simulink model "small_test"  (R2014b)
settings: Solver=FixedStepDiscrete  SolverMode=SingleTasking  StartTime=0.0  StopTime=20e-6*2  RelTol=1e-3
PreLoadFcn:
  | userName = getenv('UserName');
  | 
  | if strcmp(userName,'Tim')
  | cd C:\MA_1\Sysgen_small_test
  | else
  | cd D:\MA_1\Sysgen_small_test
  | end
InitFcn:
  | userName = getenv('UserName');
  | 
  | if strcmp(userName,'Tim')
  | cd C:\MA_1\Sysgen_small_test
  | else
  | cd D:\MA_1\Sysgen_small_test
  | end
undefined symbols (not defined in the file): bitPerSymb, gcbh, Tb, Ts, usedSubCar, xlBlockLoadCallback
libraries: xbsIndex_r4 x56, commrandsrc2 x1, simulink x1
settings Model: Creator=Tim-UML  LastModifiedBy=Tim-UML
settings DebuggingCC: AssertControl=DisableAll
settings HardwareCC: ProdBitPerLong=64  ProdBitPerPointer=64  ProdWordSize=64  ProdHWDeviceType=Generic->64-bit Embedded Processor (LP64)  TargetHWDeviceType=32-bit Generic

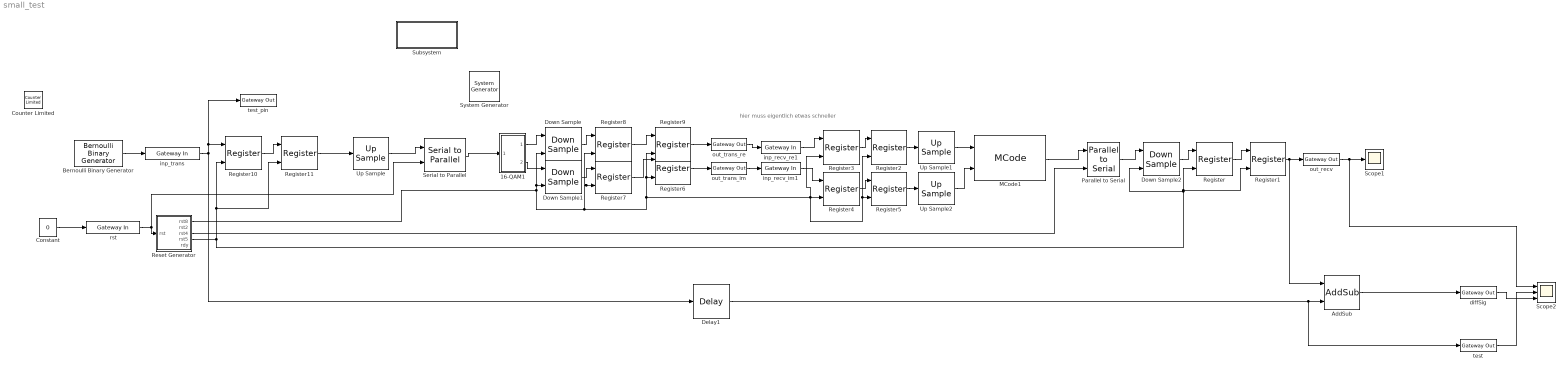
== system small_test ==
  note: hier muss eigentlich etwas schneller
  " System Generator" : xbsIndex_r4/ System Generator  Tag=genX  xilinxfamily=zynq  part=xc7z020  speed=-1  package=clg400  synthesis_tool=Vivado  clock_wrapper=Clock Enables  directory=./netlistFin3  proj_type=Vivado  Synth_file=Vivado Synthesis Defaults  Impl_file=Vivado Implementation Defaults  testbench=on  simulink_period=sysgenSystemPeriod  sysclk_period=1000/250  dcm_input_clock_period=10  incr_netlist=off  trim_vbits=Everywhere in SubSystem  dbl_ovrd=According to Block Masks  core_generation=According to Block Masks  run_coregen=off  deprecated_control=off  eval_field=0  block_type=sysgen
  16-QAM1 : Subsystem
  AddSub : xbsIndex_r4/AddSub  mode=Subtraction  use_carryin=off  use_carryout=off  en=off  latency=1  precision=User Defined  arith_type=Unsigned  n_bits=1  bin_pt=0  quantization=Truncate  overflow=Wrap  use_behavioral_HDL=off  hw_selection=Fabric  pipelined=off  dbl_ovrd=off  block_type=addsub
  Bernoulli Binary Generator : commrandsrc2/Bernoulli Binary Generator  P=0.5  seed=1604198  Ts=Tb  frameBased=off  sampPerFrame=1  orient=off  outDataType=boolean
      settings: AttributesFormatString=|
      | Sample Time= %<Ts>
      | Prob zero=%<P>
  Constant : Constant  Value=0
  Counter Limited : simulink/Sources/Counter Limited  uplimit=1  tsamp=Tb
  Delay1 : xbsIndex_r4/Delay  rst=off  infoeditControl=Selection of Reset will increase slice count due to use of real FFs and instead of SRLs  en=off  latency=14  reg_retiming=off  dbl_ovrd=off  block_type=delay
  Down Sample : xbsIndex_r4/Down Sample  sample_ratio=2  sample_phase="Last Value of Frame  (most efficient)"  en=off  rst=on  latency=1  dbl_ovrd=off  block_type=dsamp
  Down Sample1 : xbsIndex_r4/Down Sample  sample_ratio=2  sample_phase="Last Value of Frame  (most efficient)"  en=off  rst=on  latency=1  dbl_ovrd=off  block_type=dsamp
  Down Sample2 : xbsIndex_r4/Down Sample  sample_ratio=5  sample_phase="Last Value of Frame  (most efficient)"  en=off  rst=on  latency=1  dbl_ovrd=off  block_type=dsamp
  MCode1 : xbsIndex_r4/MCode  mfname=Demod_16QAM  explicit_period=off  period=1  inputsTable={'boundInpExpr'=>['',''],'inputs'=>['I','Q']}  outputsTable={'outputs'=>['y1'],'suppressOut'=>['off']}  enable_stdout=off  enable_debug=off  suppress_output=on  defparams={}  hide_port_list={}  dbl_ovrd=off  block_type=mcode
  Parallel to Serial : xbsIndex_r4/Parallel to Serial  output_order=Most Significant Word First  arith_type=Unsigned  output_bits=1  bin_pt=0  rst=on  en=off  latency=1  dbl_ovrd=off  block_type=p2s
      settings: infoedit=Each sample presented at the input becomes several samples presented serially at the output.
  Register{,1..11} (12 alike) : xbsIndex_r4/Register  init=0  rst=on  en=off  dbl_ovrd=off  block_type=register
  Reset Generator : Subsystem  LoadFcn=xlBlockLoadCallback(gcbh);  mask(Xilinx Reset Generator Block){infoedit=Captures the user's reset signal that is running at the system sample rate, and produces a downsampled reset signal running at the rates specified on the block.  The downsampled reset signals are synchronized in the same way as they are during startup.  The RDY output signal indicates when the downsampled resets are no longer asserted after the input reset is detected., rates=[5 4 2 8], previous_rates=5  4  2  8, has_advanced_control=0, sggui_pos=-1,-1,-1,-1, block_type=resetgenerator, block_version=1.0, sg_icon_stat=55,56,1,5,white,blue,0,4a55d45e49b130f2bb5565f39ca9cc33,right,,[ ],[ ], sg_mask_display=|, sg_list_contents=, sg_blockgui_xml=}
      mask sg_mask_display=|
      | fprintf('','COMMENT: begin icon graphics');
      | patch([0 55 55 0 0 ],[0 0 56 56 0 ],[0.77 0.82 0.91 ]);
      | plot([0 55 55 0 0 ],[0 0 56 56 0 ]);
      | patch([11.425 21.54 28.54 35.54 42.54 28.54 18.425 11.425 ],[35.77 35.77 42.77 35.77 42.77 42.77 42.77 35.77 ],[1 1 1 ]);
      | patch([18.425 28.54 21.54 11.425 18.425 ],[28.77 28.77 35.77 35.77 28.77 ],[0.931 0.946 0.973 ]);
      | patch([11.425 21.54 28.54 18.425 11.425 ],[21.77 21.77 28.77 28.77 21.77 ],[1 1 1 ]);
      | patch([18.425 42.54 35.54 28.54 21.54 11.425 18.425 ],[14.77 14.77 21.77 14.77 21.77 21.77 14.77 ],[0.931 0.946 0.973 ]);
      | fprintf('','COMMENT: end icon graphics');
      | fprintf('','COMMENT: begin icon text');
      | color('black');port_label('input',1,'rst');
      | color('black');port_label('output',1,'rst8');
      | color('black');port_label('output',2,'rst2');
      | color('black');port_label('output',3,'rst4');
      | color('black');port_label('output',4,'rst5');
      | color('black');port_label('output',5,'rdy');
      | fprintf('','COMMENT: end icon text');
      mask prompts: infoedit ""; rates "Specify design sample rates in MATLAB vector format, e.g. [2  4 16]"; previous_rates ""; has_advanced_control ""; sggui_pos ""; block_type ""; block_version ""; sg_icon_stat ""; sg_mask_display ""; sg_list_contents ""; sg_blockgui_xml ""
      mask help: Captures the user's reset signal that is running at the system sample rate, and produces a downsampled reset signal running at the rates specified on the block. The downsampled reset signals are synchronized in the same way as they are during startup. The RDY output signal indicates when the downsampled resets are no longer asserted after the input reset is detected.
      mask init:
      | try
      |   tmp_gcb = gcb;
      |   tmp_gcbh = gcbh;
      |   if (strcmp('SysGenIndex',get_param(bdroot(tmp_gcbh),'tag')) && ~isempty(regexp(bdroot(tmp_gcb), '^xbs', 'once')))
      |     return;
      |   end;
      |   xlMungeMaskParams;
      | 
      |   block_type='resetgenerator';
      | 
      |   serialized_declarations = '{''xinports''=>''DoubleVector'',''xoutports''=>''DoubleVector'',''block_type''=>''String''}';
      |   xlReset_init();
      |   ptable_ = xlblockprep(get_param(tmp_gcb, 'MaskWSVariables'));
      |   try
      |     xlBlockMoveCallback(tmp_gcbh);
      |   catch 
      |      clear global xl_updateicon_recursion_guard;
      |   end;
      | catch
      |   global dbgsysgen;
      |   if(~isempty(dbgsysgen) && dbgsysgen)
      |     e = regexprep(lasterr, '\n', '\nError: ');
      |     disp(['Error: While running MaskInit code on block ' tmp_gcb ': ' e]);
      |     error(e);
      |   end
      | end
      settings: CopyFcn=tmp_gcbh = gcbh;set_param(tmp_gcbh,'linkstatus','none');xlBlockMoveCallback(gcbh);  DeleteFcn=xlDestroyGui(gcbh);  ModelCloseFcn=xlDestroyGui(gcbh);  PreSaveFcn=xlBlockPreSaveCallback(gcbh);  PostSaveFcn=xlBlockPostSaveCallback(gcbh);  DestroyFcn=xlDestroyGui(gcbh);  OpenFcn=xlOpenGui(gcbh, 'xlReset_gui.xml', -1, -1)  CloseFcn=xlDestroyGui(gcbh);  MoveFcn=xlBlockMoveCallback(gcbh);
      mask Help: eval('');xlDoc('-book','sysgen','-topic','Reset_Generator');
      mask Display:
      | fprintf('','COMMENT: begin icon graphics');
      | patch([0 55 55 0 0 ],[0 0 56 56 0 ],[0.77 0.82 0.91 ]);
      | plot([0 55 55 0 0 ],[0 0 56 56 0 ]);
      | patch([11.425 21.54 28.54 35.54 42.54 28.54 18.425 11.425 ],[35.77 35.77 42.77 35.77 42.77 42.77 42.77 35.77 ],[1 1 1 ]);
      | patch([18.425 28.54 21.54 11.425 18.425 ],[28.77 28.77 35.77 35.77 28.77 ],[0.931 0.946 0.973 ]);
      | patch([11.425 21.54 28.54 18.425 11.425 ],[21.77 21.77 28.77 28.77 21.77 ],[1 1 1 ]);
      | patch([18.425 42.54 35.54 28.54 21.54 11.425 18.425 ],[14.77 14.77 21.77 14.77 21.77 21.77 14.77 ],[0.931 0.946 0.973 ]);
      | fprintf('','COMMENT: end icon graphics');
      | fprintf('','COMMENT: begin icon text');
      | color('black');port_label('input',1,'rst');
      | color('black');port_label('output',1,'rst8');
      | color('black');port_label('output',2,'rst2');
      | color('black');port_label('output',3,'rst4');
      | color('black');port_label('output',4,'rst5');
      | color('black');port_label('output',5,'rdy');
      | fprintf('','COMMENT: end icon text');
  Scope1 : Scope
      settings: TimeRange=1.102458307597285e-07  YMin=-0  YMax=2  SaveName=ScopeData92
  Scope2 : Scope  NumInputPorts=3
      settings: TimeRange=1.102458307597285e-07  YMin=-0~-5~-5  YMax=2~5~5
  Serial to Parallel : xbsIndex_r4/Serial to Parallel  input_order=Most Significant Word First  arith_type=Unsigned  output_bits=4  bin_pt=0  rst=on  en=off  latency=1  dbl_ovrd=off  block_type=s2p
      settings: infoedit=Groups of samples presented serially at the input become single samples presented at the output.
  Subsystem : Subsystem  mask(Model Parameters){upsample=No, dmtOfdm=DMT, guardInterval=Yes, AWGN=No, channel=No, equalizer=No, SampleTime=20e-9, BitTime=20e-9, modu_mode=0, radio_precision=fixpoint, bitCount=16, fracLen=13, impulseResponse=No}
      mask prompts: upsample "Enable Upsampling"; dmtOfdm "Select FFT Inputorder"; guardInterval "Guard Interval"; SampleTime "Sample Time [s]"; BitTime "Bit Time"; modu_mode "Modulation Mode"; radio_precision "Select Precision"; bitCount "Bit Count"; fracLen "Fraction Length"; impulseResponse "Measure Impulse Response"
      mask init:
      | initScript
      mask TypeOptions upsample: No | Yes
      mask TypeOptions dmtOfdm: OFDM | DMT
      mask TypeOptions guardInterval: No | Yes
      mask TypeOptions AWGN: No | Yes
      mask TypeOptions channel: No | Yes
      mask TypeOptions equalizer: No | Yes
      mask TypeOptions radio_precision: double | fixpoint
      mask TypeOptions impulseResponse: No | Yes
      mask DialogControl Container3 Prompt: Only for Fixpoint
      mask Display: disp('Edit Model\n Parameters')
  Up Sample : xbsIndex_r4/Up Sample  sample_ratio=5  copy_samples=on  en=off  latency=0  dbl_ovrd=off  block_type=usamp
  Up Sample1 : xbsIndex_r4/Up Sample  sample_ratio=2  copy_samples=on  en=off  latency=0  dbl_ovrd=off  block_type=usamp
  Up Sample2 : xbsIndex_r4/Up Sample  sample_ratio=2  copy_samples=on  en=off  latency=0  dbl_ovrd=off  block_type=usamp
  diffSig : xbsIndex_r4/Gateway Out  inherit_from_input=off  hdl_port=on  rows=1  columns=1  UseAsDAC=off  DACChannel='1'  interface=None  automatic_assignment=on  address_offset=hex2dec('00')  intf_description=''  timing_constraint=Data Rate  locs_specified=off  LOCs={}  io_standard={}  block_type=gatewayout
  inp_recv_im1 : xbsIndex_r4/Gateway In  gui_display_data_type=Fixed-point  arith_type="Signed  (2's comp)"  n_bits=16  bin_pt=fracLen  preci_type=Single  exp_width=8  frac_width=24  rows=1  columns=1  quantization="Round  (unbiased: +/- Inf)"  overflow=Saturate  period=Tb/5*8  UseAsADC=off  ADCChannel='1'  interface=None  automatic_assignment=on  address_offset=hex2dec('00')  intf_description=''  timing_constraint=None  locs_specified=off  LOCs={}  io_standard={}  inherit_from_input=off  hdl_port=on  dbl_ovrd=off  block_type=gatewayin
  inp_recv_re1 : xbsIndex_r4/Gateway In  gui_display_data_type=Fixed-point  arith_type="Signed  (2's comp)"  n_bits=16  bin_pt=fracLen  preci_type=Single  exp_width=8  frac_width=24  rows=1  columns=1  quantization="Round  (unbiased: +/- Inf)"  overflow=Saturate  period=Tb/5*8  UseAsADC=off  ADCChannel='1'  interface=None  automatic_assignment=on  address_offset=hex2dec('00')  intf_description=''  timing_constraint=None  locs_specified=off  LOCs={}  io_standard={}  inherit_from_input=off  hdl_port=on  dbl_ovrd=off  block_type=gatewayin
  inp_trans : xbsIndex_r4/Gateway In  gui_display_data_type=Fixed-point  arith_type=Unsigned  n_bits=1  bin_pt=0  preci_type=Single  exp_width=8  frac_width=24  rows=1  columns=1  quantization=Truncate  overflow=Wrap  period=Tb  UseAsADC=off  ADCChannel='1'  interface=None  automatic_assignment=on  address_offset=hex2dec('00')  intf_description=''  timing_constraint=None  locs_specified=off  LOCs={}  io_standard={}  inherit_from_input=off  hdl_port=on  dbl_ovrd=off  block_type=gatewayin
  out_recv : xbsIndex_r4/Gateway Out  inherit_from_input=off  hdl_port=on  rows=1  columns=1  UseAsDAC=off  DACChannel='1'  interface=None  automatic_assignment=on  address_offset=hex2dec('00')  intf_description=''  timing_constraint=Data Rate  locs_specified=off  LOCs={}  io_standard={}  block_type=gatewayout
  out_trans_im : xbsIndex_r4/Gateway Out  inherit_from_input=on  hdl_port=on  rows=1  columns=1  UseAsDAC=off  DACChannel='1'  interface=None  automatic_assignment=on  address_offset=hex2dec('00')  intf_description=''  timing_constraint=None  locs_specified=off  LOCs={}  io_standard={}  block_type=gatewayout
  out_trans_re : xbsIndex_r4/Gateway Out  inherit_from_input=on  hdl_port=on  rows=1  columns=1  UseAsDAC=off  DACChannel='1'  interface=None  automatic_assignment=on  address_offset=hex2dec('00')  intf_description=''  timing_constraint=None  locs_specified=off  LOCs={}  io_standard={}  block_type=gatewayout
  rst : xbsIndex_r4/Gateway In  gui_display_data_type=Boolean  arith_type=Boolean  n_bits=1  bin_pt=0  preci_type=Single  exp_width=8  frac_width=24  rows=1  columns=1  quantization=Truncate  overflow=Wrap  period=SystemPeriod  UseAsADC=off  ADCChannel='1'  interface=None  automatic_assignment=on  address_offset=hex2dec('00')  intf_description=''  timing_constraint=None  locs_specified=off  LOCs={}  io_standard={}  inherit_from_input=off  hdl_port=on  dbl_ovrd=off  block_type=gatewayin
  test : xbsIndex_r4/Gateway Out  inherit_from_input=off  hdl_port=off  rows=1  columns=1  UseAsDAC=off  DACChannel='1'  interface=None  automatic_assignment=on  address_offset=hex2dec('00')  intf_description=''  timing_constraint=Data Rate  locs_specified=off  LOCs={}  io_standard={}  block_type=gatewayout
  test_pin : xbsIndex_r4/Gateway Out  inherit_from_input=on  hdl_port=on  rows=1  columns=1  UseAsDAC=off  DACChannel='1'  interface=None  automatic_assignment=on  address_offset=hex2dec('00')  intf_description=''  timing_constraint=None  locs_specified=off  LOCs={}  io_standard={}  block_type=gatewayout
  wires:
  out_trans_re/1 -> inp_recv_re1/1
  out_trans_im/1 -> inp_recv_im1/1
  inp_recv_re1/1 -> Register3/1
  inp_recv_im1/1 -> Register4/1
  16-QAM1/1(Out2) -> Down Sample/1
  16-QAM1/2(Out3) -> Down Sample1/1
  MCode1/1 -> Parallel to Serial/1
  Parallel to Serial/1 -> Down Sample2/1
  inp_trans/1 -> test_pin/1, Register10/1, Delay1/1
  Serial to Parallel/1 -> 16-QAM1/1(In1)
  out_recv/1 -> Scope2/1, Scope1/1
  Register/1 -> Register1/1
  Register2/1 -> Up Sample1/1
  Register3/1 -> Register2/1
  Register4/1 -> Register5/1
  Register5/1 -> Up Sample2/1
  Register6/1 -> out_trans_im/1
  Register7/1 -> Register6/1
  Register8/1 -> Register9/1
  Register9/1 -> out_trans_re/1
  Register10/1 -> Register11/1
  Register11/1 -> Up Sample/1
  Up Sample/1 -> Serial to Parallel/1
  Down Sample/1 -> Register8/1
  Down Sample1/1 -> Register7/1
  Up Sample1/1 -> MCode1/1
  Up Sample2/1 -> MCode1/2
  Down Sample2/1 -> Register/1
  Bernoulli Binary Generator/1 -> inp_trans/1
  rst/1 -> Serial to Parallel/2, Reset Generator/1(rst)
  Reset Generator/1(rst8) -> Down Sample1/2, Down Sample/2, Register8/2, Register7/2, Register2/2, Register5/2, Register3/2, Register4/2, Register9/2, Register6/2
  Reset Generator/4(rst5) -> Register11/2, Register10/2, Register1/2, Register/2, Down Sample2/2
  Reset Generator/3(rst4) -> Parallel to Serial/2
  Constant/1 -> rst/1
  Delay1/1 -> test/1, AddSub/2
  Register1/1 -> out_recv/1, AddSub/1
  AddSub/1 -> diffSig/1
  test/1 -> Scope2/2
  diffSig/1 -> Scope2/3

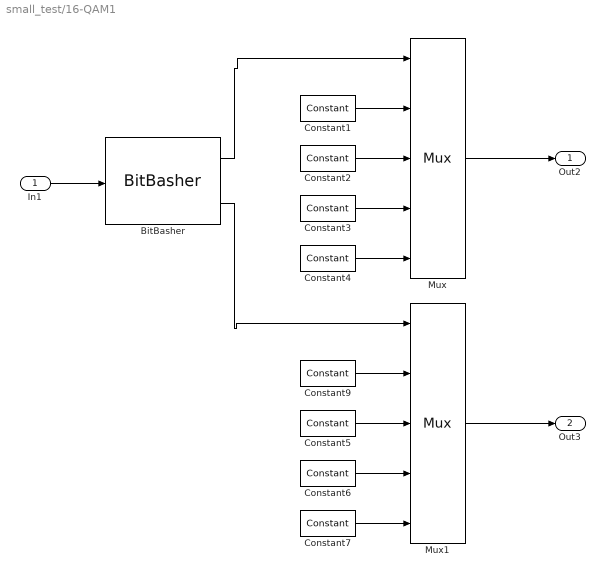
== system small_test/16-QAM1 ==
  In1 : Inport
  BitBasher : xbsIndex_r4/BitBasher  bitexpr=|  display_expr=on  sr_1=b  arith_type1=Unsigned  bin_pt1=0  sr_2=c  arith_type2=Unsigned  bin_pt2=0  sr_3=3  arith_type3=Unsigned  bin_pt3=0  sr_4=4  arith_type4=Unsigned  bin_pt4=0  dbl_ovrd=off  block_type=bitbasher
      | b={a[3:2]}
      | c={a[1:0]}
  Constant1 : xbsIndex_r4/Constant  const=-3  gui_display_data_type=Fixed-point  arith_type=Signed (2's comp)  n_bits=bitCount  bin_pt=fracLen  preci_type=Single  exp_width=8  frac_width=24  explicit_period=off  period=Ts*usedSubCar* bitPerSymb  equ=P=C  opselect=C  inp2=PCIN>>17  opr=+  inp1=P  carry=CIN  dbl_ovrd=off  block_type=constant
  Constant2 : xbsIndex_r4/Constant  const=-1  gui_display_data_type=Fixed-point  arith_type=Signed (2's comp)  n_bits=bitCount  bin_pt=fracLen  preci_type=Single  exp_width=8  frac_width=24  explicit_period=off  period=Ts*usedSubCar* bitPerSymb  equ=P=C  opselect=C  inp2=PCIN>>17  opr=+  inp1=P  carry=CIN  dbl_ovrd=off  block_type=constant
  Constant3 : xbsIndex_r4/Constant  const=3  gui_display_data_type=Fixed-point  arith_type=Signed (2's comp)  n_bits=bitCount  bin_pt=fracLen  preci_type=Single  exp_width=8  frac_width=24  explicit_period=off  period=Ts*usedSubCar* bitPerSymb  equ=P=C  opselect=C  inp2=PCIN>>17  opr=+  inp1=P  carry=CIN  dbl_ovrd=off  block_type=constant
  Constant4 : xbsIndex_r4/Constant  const=1  gui_display_data_type=Fixed-point  arith_type=Signed (2's comp)  n_bits=bitCount  bin_pt=fracLen  preci_type=Single  exp_width=8  frac_width=24  explicit_period=off  period=Ts*usedSubCar* bitPerSymb  equ=P=C  opselect=C  inp2=PCIN>>17  opr=+  inp1=P  carry=CIN  dbl_ovrd=off  block_type=constant
  Constant5 : xbsIndex_r4/Constant  const=1  gui_display_data_type=Fixed-point  arith_type=Signed (2's comp)  n_bits=bitCount  bin_pt=fracLen  preci_type=Single  exp_width=8  frac_width=24  explicit_period=off  period=Ts*usedSubCar* bitPerSymb  equ=P=C  opselect=C  inp2=PCIN>>17  opr=+  inp1=P  carry=CIN  dbl_ovrd=off  block_type=constant
  Constant6 : xbsIndex_r4/Constant  const=-3  gui_display_data_type=Fixed-point  arith_type=Signed (2's comp)  n_bits=bitCount  bin_pt=fracLen  preci_type=Single  exp_width=8  frac_width=24  explicit_period=off  period=Ts*usedSubCar* bitPerSymb  equ=P=C  opselect=C  inp2=PCIN>>17  opr=+  inp1=P  carry=CIN  dbl_ovrd=off  block_type=constant
  Constant7 : xbsIndex_r4/Constant  const=-1  gui_display_data_type=Fixed-point  arith_type=Signed (2's comp)  n_bits=bitCount  bin_pt=fracLen  preci_type=Single  exp_width=8  frac_width=24  explicit_period=off  period=Ts*usedSubCar* bitPerSymb  equ=P=C  opselect=C  inp2=PCIN>>17  opr=+  inp1=P  carry=CIN  dbl_ovrd=off  block_type=constant
  Constant9 : xbsIndex_r4/Constant  const=3  gui_display_data_type=Fixed-point  arith_type=Signed (2's comp)  n_bits=bitCount  bin_pt=fracLen  preci_type=Single  exp_width=8  frac_width=24  explicit_period=off  period=Ts*usedSubCar* bitPerSymb  equ=P=C  opselect=C  inp2=PCIN>>17  opr=+  inp1=P  carry=CIN  dbl_ovrd=off  block_type=constant
  Mux : xbsIndex_r4/Mux  inputs=4  en=off  latency=1  precision=Full  arith_type=Unsigned  n_bits=16  bin_pt=14  quantization=Truncate  overflow=Wrap  dbl_ovrd=off  block_type=mux
  Mux1 : xbsIndex_r4/Mux  inputs=4  en=off  latency=1  precision=Full  arith_type=Unsigned  n_bits=16  bin_pt=14  quantization=Truncate  overflow=Wrap  dbl_ovrd=off  block_type=mux
  Out2 : Outport
  Out3 : Outport  Port=2
  wires:
  Mux1/1 -> Out3/1
  In1/1 -> BitBasher/1
  Constant1/1 -> Mux/2
  Constant2/1 -> Mux/3
  BitBasher/1 -> Mux/1
  Constant9/1 -> Mux1/2
  Constant5/1 -> Mux1/3
  Constant7/1 -> Mux1/5
  Constant6/1 -> Mux1/4
  BitBasher/2 -> Mux1/1
  Constant4/1 -> Mux/5
  Mux/1 -> Out2/1
  Constant3/1 -> Mux/4

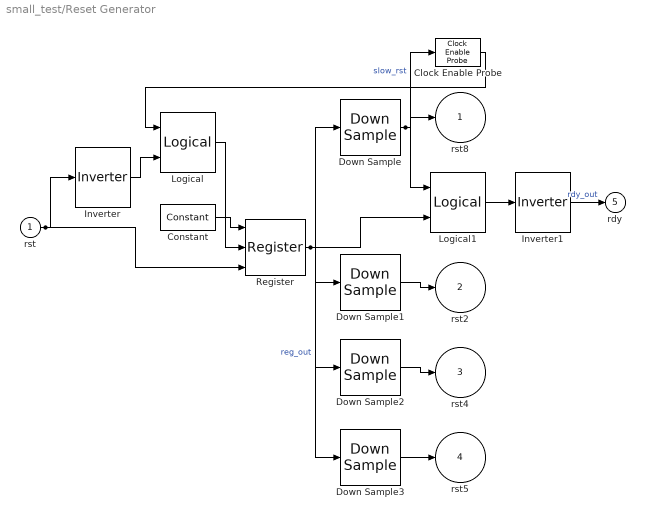
== system small_test/Reset Generator ==
  rst : Inport
  Clock Enable Probe : xbsIndex_r4/Clock Enable Probe  inherit_constraints=on  block_type=ceprobe
      settings: infoedit="Clock enable extractor.  Produces a Boolean output that mirrors the hardware clock enable associated with the input sample rate.<br><br>Hardware notes: in hardware this block costs nothing."
  Constant : xbsIndex_r4/Constant  const=1  gui_display_data_type=Fixed-point  arith_type=Boolean  n_bits=1  bin_pt=0  preci_type=Single  exp_width=8  frac_width=24  explicit_period=off  period=1  equ=P=C  opselect=C  inp2=PCIN>>17  opr=+  inp1=P  carry=CIN  dbl_ovrd=off  block_type=constant
  Down Sample : xbsIndex_r4/Down Sample  sample_ratio=8  sample_phase="Last Value of Frame  (most efficient)"  en=off  rst=off  latency=1  dbl_ovrd=off  block_type=dsamp
  Down Sample1 : xbsIndex_r4/Down Sample  sample_ratio=2  sample_phase="Last Value of Frame  (most efficient)"  en=off  rst=off  latency=6  dbl_ovrd=off  block_type=dsamp
  Down Sample2 : xbsIndex_r4/Down Sample  sample_ratio=4  sample_phase="Last Value of Frame  (most efficient)"  en=off  rst=off  latency=4  dbl_ovrd=off  block_type=dsamp
  Down Sample3 : xbsIndex_r4/Down Sample  sample_ratio=5  sample_phase="Last Value of Frame  (most efficient)"  en=off  rst=off  latency=3  dbl_ovrd=off  block_type=dsamp
  Inverter : xbsIndex_r4/Inverter  en=off  latency=1  dbl_ovrd=off  block_type=inv
  Inverter1 : xbsIndex_r4/Inverter  en=off  latency=1  dbl_ovrd=off  block_type=inv
  Logical : xbsIndex_r4/Logical  logical_function=AND  inputs=2  en=off  latency=1  precision=Full  arith_type=Unsigned  n_bits=16  bin_pt=0  align_bp=on  dbl_ovrd=off  block_type=logical
  Logical1 : xbsIndex_r4/Logical  logical_function=OR  inputs=2  en=off  latency=1  precision=Full  arith_type=Unsigned  n_bits=16  bin_pt=0  align_bp=on  dbl_ovrd=off  block_type=logical
  Register : xbsIndex_r4/Register  init=0  rst=on  en=on  dbl_ovrd=off  block_type=register
  rst8 : Outport
  rst2 : Outport  Port=2
  rst4 : Outport  Port=3
  rst5 : Outport  Port=4
  rdy : Outport  Port=5
  wires:
  Down Sample/1 -> rst8/1, Logical1/1, Clock Enable Probe/1  "slow_rst"
  rst/1 -> Register/3, Inverter/1
  Register/1 -> Down Sample3/1, Down Sample2/1, Down Sample1/1, Logical1/2, Down Sample/1  "reg_out"
  Inverter1/1 -> rdy/1  "rdy_out"
  Down Sample3/1 -> rst5/1
  Down Sample2/1 -> rst4/1
  Down Sample1/1 -> rst2/1
  Logical1/1 -> Inverter1/1
  Logical/1 -> Register/2
  Constant/1 -> Register/1
  Inverter/1 -> Logical/2
  Clock Enable Probe/1 -> Logical/1

== system small_test/Subsystem ==
